simulink model "Main_bikesim_backup"  (R2025a)
settings: Solver=FixedStepAuto  StartTime=0.0  StopTime=inf  FixedStep=0.0005
values from neighbouring files (symbols this model uses):
  A_d = permute(A_d,[1,3,2])    [Main_sim.m]    (also in Startup_labview_v2.m; sensor_error_test_sequence.m = (eye(size(A))+Ts*A))
  Ad_t = eye(1)+Ts*A_t    [Main_sim.m]    (also in Startup_labview_v2.m = (eye(size(A_t))+Ts*A_t))
  B_d = zeros(V_n,7,1)    [Main_sim.m]    (also in Startup_labview_v2.m; sensor_error_test_sequence.m = Ts*B)
  badGPS = 0    [Main_sim.m]
  Bd_t = B_t*Ts    [Main_sim.m]    (also in Startup_labview_v2.m)
  bike_model = 1    [Main_sim.m]
  bike_params = LoadBikeParameters(bike)    [Compare_real_to_sim.m]    (also in MPC_Data_train.m = LoadBikeParameters("green"); Main_sim.m; Startup_labview_v2.m; sensor_error_test_sequence.m)
  C = mpc_outer_params.Cd    [MPC_Data_train.m]    (also in Main_sim.m = permute(C,[1,3,2]); Startup_labview_v2.m = permute(C,[1,3,2]); fromIMU2trajectory.m = (W_roll * W_roll.') / max(1, size(W_roll,2)); sensor_data_check.m = (W_roll * W_roll.') / max(1, size(W_roll,2)))
  C_t = zeros(V_n,1)    [Main_sim.m]    (also in Startup_labview_v2.m)
  counter = zeros(V_n,1)    [Main_sim.m]    (also in Startup_labview_v2.m; sensor_error_test_sequence.m = 9)
  D = mpc_outer_params.Dd    [MPC_Data_train.m]    (also in Main_sim.m = zeros(V_n,7,1); Startup_labview_v2.m = zeros(V_n,7,1))
  D_t = zeros(V_n,1)    [Main_sim.m]    (also in Startup_labview_v2.m)
  e1_max = abs(-k2*e2_max/k1)    [Startup_labview_v2.m]
  friction_coefficient = 0.004    [Main_sim.m]
  gg = 9.81    [Main_sim.m]    (also in Startup_labview_v2.m)
  hor_dis = 5    [Main_sim.m]
  I_balancing_outer = 0.0    (= 0)    [Main_sim.m]    (also in Startup_labview_v2.m; sensor_error_test_sequence.m)
  indoor = 0    [Main_sim.m]
  initial_state_estimate = initial_state    [Main_sim.m]    (also in sensor_error_test_sequence.m)
  interpolation = 0    [Main_sim.m]
  k1 = K(1)    [Startup_labview_v2.m]
  k2 = K(2)    [Startup_labview_v2.m]
  K_GPS = permute(K_GPS,[1,3,2])    [Main_sim.m]    (also in Startup_labview_v2.m)
  K_noGPS = permute(K_noGPS,[1,3,2])    [Main_sim.m]    (also in Startup_labview_v2.m)
  mpc_outer_params =     [MPC_params_train.mat]    (also in Main_sim.m = struct(); mpc_outer_params.mat)
  P_balancing_inner = 3.5    [Main_sim.m]    (also in Startup_labview_v2.m; sensor_error_test_sequence.m)
  P_balancing_outer = 3.75    [Main_sim.m]    (also in Startup_labview_v2.m; sensor_error_test_sequence.m)
  Psiref = [Psiref(1); Psiref]    [ReferenceGenerator.m]    (also in differenttest.m = [atan2(Yref(2)-Yref(1), Xref(2)-Xref(1)); differenttest_Simon.m = [psi(1); psi])
  ref_dis = 1    [Main_sim.m]    (also in differenttest.m = 0.1; differenttest_Simon.m = 0.1)
  T = [ 1,  sin(phi)*tan(th),  cos(phi)*tan(th) ... (first row only)    [Copy_of_fromIMU2trajectory.m]    (also in Main_sim.m = TransMatrix(bike_params); fromIMU2trajectory.m; sensor_error_test_sequence.m = Rz*Ry*Rx; shorttrajectory.m = table(Xref, Yref, Psiref, Vref, t, 'VariableNames', {'Xref',)
  t_ref = linspace(0, (lL-1)/Vref_test, lL)'    [differenttest.m]    (also in differenttest_Simon.m)
  Ts = 0.01    [Main_sim.m]    (also in Startup_labview_v2.m; sensor_error_test_sequence.m)
  V = round(V,1)    [Main_sim.m]    (also in Startup_labview_v2.m)
  v_init = Vref(1)    [Main_sim.m]    (also in Startup_labview_v2.m)
  Vref = zeros(length(Xref), 1)    [Refgeneration_test.m]    (also in differenttest_Simon.m = Vref_test * ones(N_line, 1))
  vv = 2    [Main_sim.m]    (also in Refgeneration.m = table_ref.v)
  Xref = [Xref;Xref2]    [ReferenceGenerator.m]    (also in concatenate.m; differenttest.m = interp1(cumulative_distance, x, equal_distances)'; differenttest_Simon.m = interp1(s, x_path, s_eq, 'linear')')
  Yref = [Yref;Yref2]    [ReferenceGenerator.m]    (also in concatenate.m; differenttest.m = interp1(cumulative_distance, y, equal_distances)'; differenttest_Simon.m = interp1(s, y_path, s_eq, 'linear')')
undefined symbols (not defined in the file or in its folder): initial_state, MPC_Ts, pert_deltadot_state, pert_deltadot_state_fun, pert_phidot_state, pert_phidot_state_fun
libraries: simulink x10, slpidlib x4, matrix_library x1, eeGeneralControl x1
(part 2 of 3)

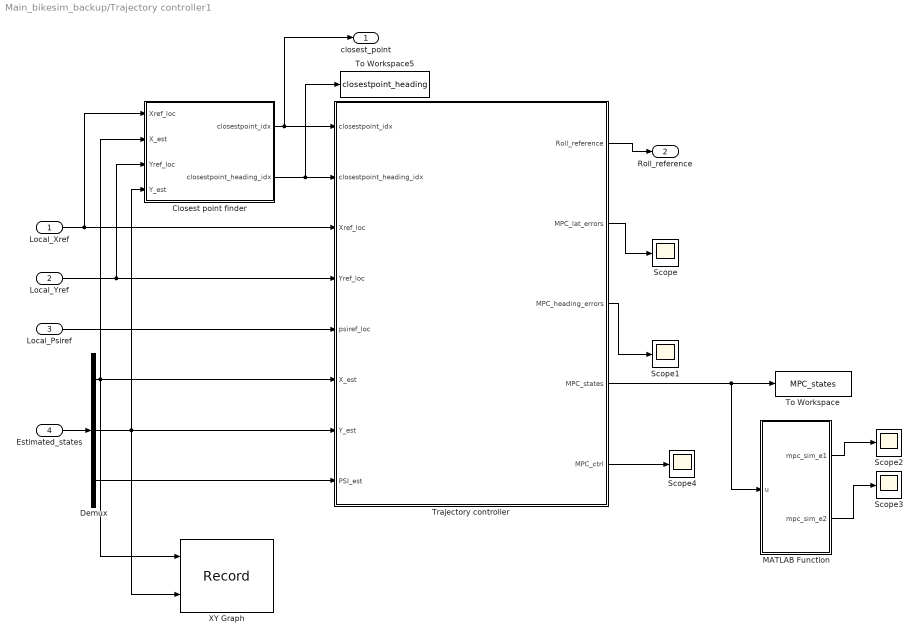
== system Main_bikesim_backup/Trajectory controller1 ==
  Local_Xref : Inport
  Local_Yref : Inport  Port=2
  Local_Psiref : Inport  Port=3
  Estimated_states : Inport  Port=4
  Closest point finder : MATLAB Function  TreatAsAtomicUnit=on
  Demux : Demux  Outputs=3
  MATLAB Function : MATLAB Function  TreatAsAtomicUnit=on
  Scope{,1..4} (5 alike) : Scope
      Scope settings: ActiveDisplayYMinimum=-10.323052116626126  ActiveDisplayYMaximum=2.50520359067044  DataLoggingVariableName=ScopeData21
      Scope1 settings: ActiveDisplayYMinimum=-2.3069490270114361  ActiveDisplayYMaximum=0.25967766677403764  DataLoggingVariableName=ScopeData22
      Scope2 settings: ActiveDisplayYMinimum=-0.54382498124419365  ActiveDisplayYMaximum=0.057362051727919812  DataLoggingVariableName=ScopeData28
      Scope3 settings: ActiveDisplayYMinimum=-0.21677334939399687  ActiveDisplayYMaximum=0.018061249921101648  DataLoggingVariableName=ScopeData29
      Scope4 settings: ActiveDisplayYMinimum=-0.43633231299858333  ActiveDisplayYMaximum=0.436332312998583  DataLoggingVariableName=ScopeData30
  To Workspace : ToWorkspace  VariableName=MPC_states  SaveFormat=Timeseries  SampleTime=-1
  To Workspace5 : ToWorkspace  VariableName=closestpoint_heading  SaveFormat=Timeseries  SampleTime=-1
  Trajectory controller : MATLAB Function  TreatAsAtomicUnit=on
  XY Graph : Record  NumPorts=2.0  FileSettingsInternal="{\"entries\":[{\"content\":{\"excelSettings\":{\"content\":{},\"type\":\"Streamout.ExcelSettings\"},\"parquetSettings\":{\"content\":{},\"type\":\"Streamout.ParquetSettings\"}},\"type\":\"Streamout.FileSettingStorage\",\"uuid\":\"\"}],\"packageUris\":[\"http:\\/\\/schema.mathworks.com\\/mf0\\/streamout_blocks\\/R2020a\"],\"version\":\"1.0\"}"  FrameSettings=[0, 0]  Layout=[1 1]  SignalsInternal="{\"entries\":[{\"content\":{\"signals\":[{\"content\":{\"blockPath\":[],\"dimensions\":[1],\"domain\":\"\",\"lineColor\":\"#edb120\",\"lineWidth\":2,\"port\":1,\"sid\":[\"\"],\"signalID\":1},\"type\":\"RecordBlkView.Signal\",\"uuid\":\"\"},{\"content\":{\"blockPath\":[],\"dimensions\":[1],\"domain\":\"\",\"lineColor\":\"#7e2f8e\",\"lineWidth\":2,\"port\":1,\"sid\":[\"\"],\"signalID\":2,\"signalName\":\"Add\"},\"type\":\"RecordBlkView.Signal\",\"uuid\":\"\"},{\"content\":{\"blockPath\":[],\"dimensions\":[7],\"domain\":\"\",\"hasChildren\":true,\"lineColor\":\"#7e2f8e\",\"lineWidth\":2,\"port\":1,\"sid\":[\"\"],\"signalID\":3},\"type\":\"RecordBlkView.Signal\",\"uuid\":\"\"},{\"content\":{\"blockPath\":[],\"channel\":[1],\"dimensions\":[7],\"domain\":\"\",\"lineColor\":\"#4dbeee\",\"lineWidth\":2,\"parentID\":3,\"port\":1,\"sid\":[\"\"],\"signalID\":4},\"type\":\"RecordBlkView.Signal\",\"uuid\":\"\"},{\"content\":{\"blockPath\":[],\"dimensions\":[1],\"domain\":\"\",\"lineColor\":\"#a2142f\",\"lineWidth\":2,\"port\":1,\"sid\":[\"\"],\"signalID\":5,\"signalName\":\"calculate pose_error based on projection point to reference point at time t\"},\"type\":\"RecordBlkView.Signal\",\"uuid\":\"\"},{\"content\":{\"blockPath\":[],\"dimensions\":[1],\"domain\":\"\",\"lineColor\":\"#139fff\",\"lineWidth\":2,\"port\":1,\"sid\":[\"\"],\"signalID\":6,\"signalName\":\"closest_point\"},\"type\":\"RecordBlkView.Signal\",\"uuid\":\"\"},{\"content\":{\"blockPath\":[],\"dimensions\":[7],\"domain\":\"\",\"hasChildren\":true,\"lineColor\":\"#139fff\",\"lineWidth\":2,\"port\":1,\"sid\":[\"\"],\"signalID\":7},\"type\":\"RecordBlkView.Signal\",\"uuid\":\"\"},{\"content\":{\"blockPath\":[],\"channel\":[1],\"dimensions\":[7],\"domain\":\"\",\"lineColor\":\"#b746ff\",\"lineWidth\":2,\"parentID\":7,\"port\":1,\"sid\":[\"\"],\"signalID\":8},\"type\":\"RecordBlkView.Signal\",\"uuid\":\"\"},{\"content\":{\"blockPath\":[],\"dimensions\":[7],\"domain\":\"\",\"hasChildren\":true,\"lineColor\":\"#b746ff\",\"lineWidth\":2,\"port\":1,\"sid\":[\"\"],\"signalID\":9},\"type\":\"RecordBlkView.Signal\",\"uuid\":\"\"},{\"content\":{\"blockPath\":[],\"channel\":[1],\"dimensions\":[7],\"domain\":\"\",\"lineColor\":\"#ff13a6\",\"lineWidth\":2,\"parentID\":9,\"port\":1,\"sid\":[\"\"],\"signalID\":10},\"type\":\"RecordBlkView.Signal\",\"uuid\":\"\"},{\"content\":{\"blockPath\":[],\"dimensions\":[1],\"domain\":\"\",\"lineColor\":\"#7e2f8e\",\"lineWidth\":2,\"port\":1,\"sid\":[\"\"],\"signalID\":11,\"signalName\":\"Trajectory controller:1\"},\"type\":\"RecordBlkView.Signal\",\"uuid\":\"\"},{\"content\":{\"blockPath\":[],\"dimensions\":[1],\"domain\":\"\",\"lineColor\":\"#77ac30\",\"lineWidth\":2,\"port\":1,\"sid\":[\"\"],\"signalID\":12,\"signalName\":\"Trajectory controller:2\"},\"type\":\"RecordBlkView.Signal\",\"uuid\":\"\"},{\"content\":{\"blockPath\":[],\"dimensions\":[1],\"domain\":\"\",\"lineColor\":\"#4dbeee\",\"lineWidth\":2,\"port\":1,\"sid\":[\"\"],\"signalID\":13,\"signalName\":\"Trajectory controller:6\"},\"type\":\"RecordBlkView.Signal\",\"uuid\":\"\"},{\"content\":{\"blockPath\":[],\"dimensions\":[1],\"domain\":\"\",\"lineColor\":\"#a2142f\",\"plots\":[ 1 ],\"port\":1,\"sid\":[\"\"],\"signalID\":14,\"signalName\":\"Demux:1\"},\"type\":\"RecordBlkView.Signal\",\"uuid\":\"\"},{\"content\":{\"blockPath\":[],\"dimensions\":[1],\"domain\":\"\",\"lineColor\":\"#139fff\",\"plots\":[ 1 ],\"port\":2,\"sid\":[\"\"],\"signalID\":15,\"signalName\":\"Demux:2\"},\"type\":\"RecordBlkView.Signal\",\"uuid\":\"\"},{\"content\":{\"blockPath\":[],\"dimensions\":[260],\"domain\":\"\",\"hasChildren\":true,\"lineColor\":\"#edb120\",\"lineWidth\":2,\"port\":1,\"sid\":[\"\"],\"signalID\":16,\"signalName\":\"Trajectory controller:4\"},\"type\":\"RecordBlkView.Signal\",\"uuid\":\"\"},{\"content\":{\"blockPath\":[],\"channel\":[1],\"dimensions\":[260],\"domain\":\"\",\"lineColor\":\"#d95319\",\"lineWidth\":2,\"parentID\":16,\"port\":1,\"sid\":[\"\"],\"signalID\":17,\"signalName\":\"Trajectory controller:4\"},\"type\":\"RecordBlkView.Signal\",\"uuid\":\"\"},{\"content\":{\"blockPath\":[],\"dimensions\":[1],\"domain\":\"\",\"lineColor\":\"#edb120\",\"lineWidth\":2,\"port\":1,\"sid\":[\"\"],\"signalID\":18,\"signalName\":\"Closest point finder:2\"},\"type\":\"RecordBlkView.Signal\",\"uuid\":\"\"},{\"content\":{\"blockPath\":[],\"dimensions\":[1],\"domain\":\"\",\"lineColor\":\"#7e2f8e\",\"lineWidth\":2,\"port\":1,\"sid\":[\"\"],\"signalID\":19},\"type\":\"RecordBlkView.Signal\",\"uuid\":\"\"},{\"content\":{\"blockPath\":[],\"dimensions\":[7],\"domain\":\"\",\"hasChildren\":true,\"lineColor\":\"#a2142f\",\"lineWidth\":2,\"port\":1,\"sid\":[\"\"],\"signalID\":20,\"signalName\":\"Mux\"},\"type\":\"RecordBlkView.Signal\",\"uuid\":\"\"},{\"content\":{\"blockPath\":[],\"channel\":[1],\"dimensions\":[7],\"domain\":\"\",\"lineColor\":\"#4dbeee\",\"lineWidth\":2,\"parentID\":20,\"port\":1,\"sid\":[\"\"],\"signalID\":21,\"signalName\":\"Mux\"},\"type\":\"RecordBlkView.Signal\",\"uuid\":\"\"},{\"content\":{\"blockPath\":[],\"dimensions\":[7],\"domain\":\"\",\"hasChildren\":true,\"lineColor\":\"#ff6929\",\"lineWidth\":2,\"port\":1,\"sid\":[\"\"],\"signalID\":22,\"signalName\":\"From10\"},\"type\":\"RecordBlkView.Signal\",\"uuid\":\"\"},{\"content\":{\"blockPath\":[],\"channel\":[1],\"dimensions\":[7],\"domain\":\"\",\"lineColor\":\"#139fff\",\"lineWidth\":2,\"parentID\":22,\"port\":1,\"sid\":[\"\"],\"signalID\":23,\"signalName\":\"From10\"},\"type\":\"RecordBlkView.Signal\",\"uuid\":\"\"},{\"content\":{\"blockPath\":[],\"dimensions\":[1],\"domain\":\"\",\"lineColor\":\"#a2142f\",\"lineWidth\":2,\"port\":1,\"sid\":[\"\"],\"signalID\":24,\"signalName\":\"From11\"},\"type\":\"RecordBlkView.Signal\",\"uuid\":\"\"},{\"content\":{\"blockPath\":[],\"dimensions\":[1],\"domain\":\"\",\"lineColor\":\"#139fff\",\"lineWidth\":2,\"port\":1,\"sid\":[\"\"],\"signalID\":25,\"signalName\":\"From12\"},\"type\":\"RecordBlkView.Signal\",\"uuid\":\"\"},{\"content\":{\"blockPath\":[],\"dimensions\":[1],\"domain\":\"\",\"lineColor\":\"#ff6929\",\"lineWidth\":2,\"port\":1,\"sid\":[\"\"],\"signalID\":26,\"signalName\":\"From13\"},\"type\":\"RecordBlkView.Signal\",\"uuid\":\"\"},{\"content\":{\"blockPath\":[],\"dimensions\":[1],\"domain\":\"\",\"lineColor\":\"#ff6929\",\"lineWidth\":2,\"port\":1,\"sid\":[\"\"],\"signalID\":27,\"signalName\":\"From17\"},\"type\":\"RecordBlkView.Signal\",\"uuid\":\"\"},{\"content\":{\"blockPath\":[],\"dimensions\":[1],\"domain\":\"\",\"lineColor\":\"#b746ff\",\"lineWidth\":2,\"port\":1,\"sid\":[\"\"],\"signalID\":28,\"signalName\":\"From18\"},\"type\":\"RecordBlkView.Signal\",\"uuid\":\"\"},{\"content\":{\"blockPath\":[],\"dimensions\":[1],\"domain\":\"\",\"lineColor\":\"#64d413\",\"lineWidth\":2,\"port\":1,\"sid\":[\"\"],\"signalID\":29,\"signalName\":\"From19\"},\"type\":\"RecordBlkView.Signal\",\"uuid\":\"\"},{\"content\":{\"blockPath\":[],\"dimensions\":[1],\"domain\":\"\",\"lineColor\":\"#ff13a6\",\"lineWidth\":2,\"port\":1,\"sid\":[\"\"],\"signalID\":30,\"signalName\":\"From20\"},\"type\":\"RecordBlkView.Signal\",\"uuid\":\"\"},{\"content\":{\"blockPath\":[],\"dimensions\":[20],\"domain\":\"\",\"lineColor\":\"#fe330a\",\"lineWidth\":2,\"port\":1,\"sid\":[\"\"],\"signalID\":31,\"signalName\":\"From21\"},\"type\":\"RecordBlkView.Signal\",\"uuid\":\"\"},{\"content\":{\"blockPath\":[],\"dimensions\":[20],\"domain\":\"\",\"lineColor\":\"#22b573\",\"lineWidth\":2,\"port\":1,\"sid\":[\"\"],\"signalID\":32,\"signalName\":\"From22\"},\"type\":\"RecordBlkView.Signal\",\"uuid\":\"\"},{\"content\":{\"blockPath\":[],\"dimensions\":[1],\"domain\":\"\",\"lineColor\":\"#0072bd\",\"lineWidth\":2,\"port\":1,\"sid\":[\"\"],\"signalID\":33,\"signalName\":\"From5\"},\"type\":\"RecordBlkView.Signal\",\"uuid\":\"\"},{\"content\":{\"blockPath\":[],\"dimensions\":[7],\"domain\":\"\",\"hasChildren\":true,\"lineColor\":\"#a2142f\",\"lineWidth\":2,\"port\":1,\"sid\":[\"\"],\"signalID\":34,\"signalName\":\"From7\"},\"type\":\"RecordBlkView.Signal\",\"uuid\":\"\"},{\"content\":{\"blockPath\":[],\"channel\":[1],\"dimensions\":[7],\"domain\":\"\",\"lineColor\":\"#edb120\",\"lineWidth\":2,\"parentID\":34,\"port\":1,\"sid\":[\"\"],\"signalID\":35,\"signalName\":\"From7\"},\"type\":\"RecordBlkView.Signal\",\"uuid\":\"\"},{\"content\":{\"blockPath\":[],\"dimensions\":[7],\"domain\":\"\",\"hasChildren\":true,\"lineColor\":\"#ff6929\",\"lineWidth\":2,\"port\":1,\"sid\":[\"\"],\"signalID\":36,\"signalName\":\"From8\"},\"type\":\"RecordBlkView.Signal\",\"uuid\":\"\"},{\"content\":{\"blockPath\":[],\"channel\":[1],\"dimensions\":[7],\"domain\":\"\",\"lineColor\":\"#77ac30\",\"lineWidth\":2,\"parentID\":36,\"port\":1,\"sid\":[\"\"],\"signalID\":37,\"signalName\":\"From8\"},\"type\":\"RecordBlkView.Signal\",\"uuid\":\"\"},{\"content\":{\"blockPath\":[],\"dimensions\":[1],\"domain\":\"\",\"lineColor\":\"#4dbeee\",\"lineWidth\":2,\"port\":1,\"sid\":[\"\"],\"signalID\":38,\"signalName\":\"From9\"},\"type\":\"RecordBlkView.Signal\",\"uuid\":\"\"}]},\"type\":\"RecordBlkView.InputSignals\",\"uuid\":\"\"}],\"packageUris\":[\"http:\\/\\/schema.mathworks.com\\/mf0\\/streamout_blocks\\/R2020a\"],\"version\":\"1.0\"}"  VisualizationBindings="{\"xyplotplugin\":{\"info\":[{\"series\":[{\"bindingParametersList\":[{\"parameter\":\"X-Axis\",\"signalID\":14,\"signalName\":\"Demux:1\"},{\"parameter\":\"Y-Axis\",\"signalID\":15,\"signalName\":\"Demux:2\"}],\"seriesID\":0}],\"subplotID\":1}]}}"  CompatibilityTag=XY
  closest_point : Outport
  Roll_reference : Outport  Port=2
  wires:
  Estimated_states/1 -> Demux/1
  Local_Xref/1 -> Closest point finder/1(Xref_loc), Trajectory controller/3(Xref_loc)
  Local_Psiref/1 -> Trajectory controller/5(psiref_loc)
  Demux/2 -> XY Graph/2, Closest point finder/4(Y_est), Trajectory controller/7(Y_est)
  Local_Yref/1 -> Closest point finder/3(Yref_loc), Trajectory controller/4(Yref_loc)
  Demux/1 -> XY Graph/1, Closest point finder/2(X_est), Trajectory controller/6(X_est)
  Closest point finder/1(closestpoint_idx) -> closest_point/1, Trajectory controller/1(closestpoint_idx)
  Closest point finder/2(closestpoint_heading_idx) -> To Workspace5/1, Trajectory controller/2(closestpoint_heading_idx)
  Demux/3 -> Trajectory controller/8(PSI_est)
  Trajectory controller/2(MPC_lat_errors) -> Scope/1
  Trajectory controller/3(MPC_heading_errors) -> Scope1/1
  Trajectory controller/1(Roll_reference) -> Roll_reference/1
  Trajectory controller/4(MPC_states) -> MATLAB Function/1(u), To Workspace/1
  MATLAB Function/1(mpc_sim_e1) -> Scope2/1
  MATLAB Function/2(mpc_sim_e2) -> Scope3/1
  Trajectory controller/5(MPC_ctrl) -> Scope4/1

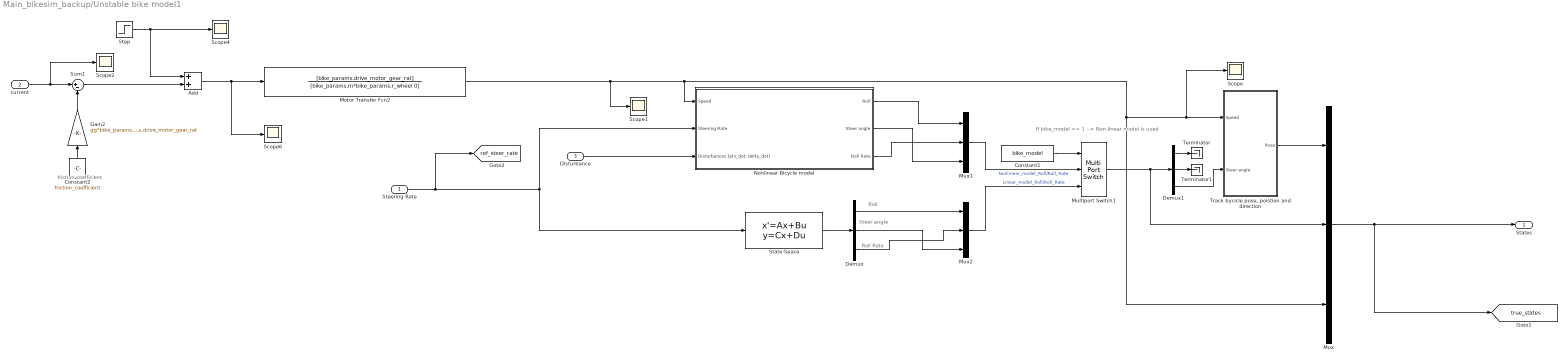
== system Main_bikesim_backup/Unstable bike model1 ==
  note: Steer angle
  note: Roll Rate
  note: Roll
  note: If bike_model == 1 --> Non-linear model is used
  note: friction coefficient
  Steering Rate : Inport
  current : Inport  Port=2
  Disturbance : Inport  Port=3
  Add : Sum
  Constant1 : Constant  Value=bike_model
  Constant2 : Constant  Value=friction_coefficient
  Demux : Demux  Outputs=3
  Demux1 : Demux  Outputs=3
  Gain2 : Gain  Gain=gg*bike_params.m*bike_params.r_wheel/bike_params.drive_motor_gear_rat
  Motor Transfer Fcn2 : TransferFcn  Numerator=[bike_params.drive_motor_gear_rat]  Denominator=[bike_params.m*bike_params.r_wheel 0]
  Multiport Switch1 : MultiPortSwitch  Inputs=2  SaturateOnIntegerOverflow=off  InputSameDT=off
  Mux : Mux  Inputs=3
  Mux1 : Mux  Inputs=3
  Mux2 : Mux  Inputs=3
  Nonlinear Bicycle model : Subsystem
  Scope{,1..2,4,6} (5 alike) : Scope
      Scope settings: ActiveDisplayYMinimum=-14.800391636195144  ActiveDisplayYMaximum=2.1206123892114217  DataLoggingVariableName=ScopeData4
      Scope1 settings: ActiveDisplayYMinimum=1  ActiveDisplayYMaximum=3  DataLoggingVariableName=ScopeData2
      Scope2 settings: ActiveDisplayYMinimum=-107.24515658734754  ActiveDisplayYMaximum=16.580853648483561  DataLoggingVariableName=ScopeData3
      Scope4 settings: ActiveDisplayYMinimum=-0.125  ActiveDisplayYMaximum=1.125  DataLoggingVariableName=ScopeData5
      Scope6 settings: ActiveDisplayYMinimum=-107.26411377256493  ActiveDisplayYMaximum=16.561896463266169
  State-Space : StateSpace  A=[0 0 1; 0 0 0 ; gg/bike_params.h (vv^2/bike_params.h-(gg*bike_params.lr*bike_params.c/(bike_params.h^2*(bike_params.lr+bike_params.lf))))*sin(bike_params.lambda) 0]  B=[0; 1 ; bike_params.lr*vv/((bike_params.lr+bike_params.lf)*bike_params.h)]  C=[1 0 0; 0 1 0 ; 0 0 1]  D=[0;0;0]  InitialCondition=[0; 0 ; 0]
  Step : Step  Time=10  After=0  SampleTime=5
  Sum1 : Sum  Inputs=|+-
  Terminator : Terminator
  Terminator1 : Terminator
  "Track bycicle pose, poistion and direction" : Subsystem
  States : Outport
  tag scope: ref_steer_rate=global, true_states=global
  wires:
  Steering Rate/1 -> State-Space/1, Nonlinear Bicycle model/2(Steering Rate), [ref_steer_rate]
  Nonlinear Bicycle model/3(Roll Rate) -> Mux1/2
  Nonlinear Bicycle model/2(Steer angle) -> Mux1/3
  Demux/1 -> Mux2/1
  Demux/3 -> Mux2/2
  Mux1/1 -> Multiport Switch1/2  "Nonlinear_model_Roll/Roll_Rate"
  Mux2/1 -> Multiport Switch1/3  "Linear_model_Roll/Roll_Rate"
  Constant1/1 -> Multiport Switch1/1
  Disturbance/1 -> Nonlinear Bicycle model/3(Disturbances (phi_dot; delta_dot))
  "Track bycicle pose, poistion and direction"/1(Pose) -> Mux/1
  Mux/1 -> States/1, [true_states]
  Nonlinear Bicycle model/1(Roll) -> Mux1/1
  State-Space/1 -> Demux/1
  Demux/2 -> Mux2/3
  Multiport Switch1/1 -> Mux/2, Demux1/1
  Demux1/3 -> "Track bycicle pose, poistion and direction"/2(Steer angle)
  Demux1/1 -> Terminator/1
  Demux1/2 -> Terminator1/1
  Constant2/1 -> Gain2/1
  Gain2/1 -> Sum1/2
  Sum1/1 -> Add/2
  Motor Transfer Fcn2/1 -> Scope1/1, Mux/3, Scope/1, "Track bycicle pose, poistion and direction"/1(Speed), Nonlinear Bicycle model/1(Speed)
  Step/1 -> Add/1, Scope4/1
  current/1 -> Scope2/1, Sum1/1
  Add/1 -> Motor Transfer Fcn2/1, Scope6/1

== system Main_bikesim_backup/Sensors1/Constant disturbances ==
  note: Apply the constant noise after 8sec
  Noise Channel : Inport
  Clock : Clock
  Constant4 : Constant  Value=[1 0.5 -0.2 0.2 0.1 0.02 0.3]'
  Constant7 : Constant  Value=[ 0 0 0 0 0 0 0]
  Create Diagonal Matrix : matrix_library/Create Diagonal Matrix
      settings: LibrarySourceBlock=|
      | simulink/Matrix
      | Operations/Create Diagonal
      | Matrix
  Matrix Multiply : Product  Multiplication=Matrix(*)
  Switch : Switch  Criteria=u2 > Threshold  Threshold=8  SaturateOnIntegerOverflow=off  InputSameDT=off
  Noise : Outport
  wires:
  Create Diagonal Matrix/1 -> Matrix Multiply/1
  Constant7/1 -> Switch/3
  Matrix Multiply/1 -> Switch/1
  Clock/1 -> Switch/2
  Constant4/1 -> Matrix Multiply/2
  Switch/1 -> Noise/1
  Noise Channel/1 -> Create Diagonal Matrix/1

== system Main_bikesim_backup/Sensors1/Subsystem ==
  X_coordinate : Inport
  Clock : Clock
  Gain1 : Gain  Gain=badGPS
  Memory : Memory
  Switch : Switch  Criteria=u2 > Threshold  SaturateOnIntegerOverflow=off  InputSameDT=off
  X_coordinate from GPS : Outport
  wires:
  Memory/1 -> Switch/1
  Clock/1 -> Gain1/1
  Switch/1 -> X_coordinate from GPS/1, Memory/1
  Gain1/1 -> Switch/2
  X_coordinate/1 -> Switch/3

== system Main_bikesim_backup/Sensors1/Subsystem1 ==
  Y_coordinate : Inport
  Clock : Clock
  Gain1 : Gain  Gain=badGPS
  Memory : Memory
  Switch : Switch  Criteria=u2 > Threshold  SaturateOnIntegerOverflow=off  InputSameDT=off
  Y_coordinate from GPS : Outport
  wires:
  Y_coordinate/1 -> Switch/3
  Gain1/1 -> Switch/2
  Switch/1 -> Memory/1, Y_coordinate from GPS/1
  Clock/1 -> Gain1/1
  Memory/1 -> Switch/1

== system Main_bikesim_backup/Unstable bike model1/Nonlinear Bicycle model ==
  Speed : Inport
  Steering Rate : Inport  Port=2
  Disturbances (phi_dot; delta_dot) : Inport  Port=3
  Demux : Demux  Outputs=3
  Integrator2 : Integrator  InitialCondition=[initial_state.roll ; initial_state.steering ; initial_state.roll_rate]
  MATLAB Function : MATLAB Function  TreatAsAtomicUnit=on
  Real Bike Parameters : Constant  Value=[gg bike_params.h bike_params.lr bike_params.lf bike_params.lambda bike_params.c bike_params.m bike_params.IMU_height bike_params.Xgps bike_params.Ygps bike_params.Hgps]  SampleTime=Ts
  Roll : Outport  VectorParamsAs1DForOutWhenUnconnected=off
  Steer angle : Outport  Port=2  VectorParamsAs1DForOutWhenUnconnected=off
  Roll Rate : Outport  Port=3  VectorParamsAs1DForOutWhenUnconnected=off
  wires:
  Steering Rate/1 -> MATLAB Function/2(Steering_rate)
  Disturbances (phi_dot; delta_dot)/1 -> MATLAB Function/4(disturbances)
  Real Bike Parameters/1 -> MATLAB Function/5(bike_params)
  Speed/1 -> MATLAB Function/3(Speed)
  Demux/1 -> Roll/1  "Roll Angle"
  Demux/3 -> Roll Rate/1  "Roll Rate"
  Demux/2 -> Steer angle/1  "Steering Angle"
  Integrator2/1 -> MATLAB Function/1(States), Demux/1
  MATLAB Function/1(xdot) -> Integrator2/1

== system Main_bikesim_backup/Unstable bike model1/Track bycicle pose, poistion and direction ==
  Speed : Inport
  Steer angle : Inport  Port=2
  Constant : Constant  Value=[bike_params.lr bike_params.lf bike_params.lambda]
  Derivative of positions : MATLAB Function  TreatAsAtomicUnit=on
  Integrator with Wrapped State (between -pi & pi) : eeGeneralControl/Integrator with Wrapped State (Discrete or Continuous)  LabelModeActiveChoice=Discrete  WrappedStateUpperValue=pi  WrappedStateLowerValue=-pi  x0=initial_state_estimate.heading  Ts=Ts
  Integrator1 : Integrator  InitialCondition=initial_state_estimate.x
  Integrator2 : Integrator  InitialCondition=initial_state_estimate.y
  MATLAB Function : MATLAB Function  TreatAsAtomicUnit=on
  Mux : Mux  Inputs=3
  Pose : Outport
  tag scope: Xposition4debug=global
  wires:
  Derivative of positions/2(Ydot) -> Integrator2/1  "Ydot"
  Steer angle/1 -> MATLAB Function/2(steer_angle)
  Integrator2/1 -> Mux/2
  Mux/1 -> Pose/1
  Derivative of positions/1(Xdot) -> Integrator1/1  "Xdot"
  Speed/1 -> MATLAB Function/1(Speed), Derivative of positions/1(Speed)
  Integrator1/1 -> [Xposition4debug], Mux/1
  MATLAB Function/1(beta) -> Derivative of positions/2(beta)
  Constant/1 -> MATLAB Function/3(bike_params)
  MATLAB Function/2(psi_dot) -> Integrator with Wrapped State (between -pi & pi)/1
  Integrator with Wrapped State (between -pi & pi)/1 -> Derivative of positions/3(psi), Mux/3

== matlab function Main_bikesim_backup/current position on the trajectory, projection from estimated position ==
  settings: updateMethod=DISCRETE  sampleTime=Ts
  data: Xest input; Yest input; Xref_loc input; Yref_loc input; closest_point input; X_projection output; Y_projection output; closest2closestplus1 output
function [X_projection, Y_projection,closest2closestplus1] = Closest2estOntoClosest2interp(Xest, Yest, Xref_loc, Yref_loc, closest_point)
    
    % Construct vector closest2est
    closest2est = [Xest - Xref_loc(closest_point), Yest - Yref_loc(closest_point)];

    % Construct vector closest2closestplus1
    closest2closestplus1 = [Xref_loc(closest_point+1) - Xref_loc(closest_point), Yref_loc(closest_point+1) - Yref_loc(closest_point)];

    % Calculate the dot product of closest2est and closest2closestplus1
    dot_product = dot(closest2est, closest2closestplus1);

    % Calculate the magnitude squared of closest2closestplus1
    closest2closestplus1_magnitude_squared = dot(closest2closestplus1, closest2closestplus1);

    % Calculate the projection_ratio
    projection_ratio = dot_product/closest2closestplus1_magnitude_squared;

    % Calculate the X coordinate of the projection point
    X_projection = Xref_loc(closest_point) +  projection_ratio*(Xref_loc(closest_point+1) - Xref_loc(closest_point));

    % Calculate the Y coordinate of the projection point
    Y_projection = Yref_loc(closest_point) +  projection_ratio*(Yref_loc(closest_point+1) - Yref_loc(closest_point));
end

== matlab function Main_bikesim_backup/Sensors1/MATLAB Function ==
  data: V parameter; C3 output; C parameter; Estimated_Velocity input; interpolation parameter
function C3=fcn(V, C, Estimated_Velocity, interpolation)
% Finding the index of closest and second closest velocities in the calculated velocity vector(in main.m) that corresponds to the
% gains and matrices based on our estimated velocity (i.e the estimated
% velocity is between these two closest V's)
    differences = abs(V - Estimated_Velocity);
    [~, index1] = min(differences);
    differences(index1)=inf;
    [~, index2] = min(differences);

% Implementing linear interpolation when estimated velocity is inside the
% range of minimum and maximum calculated velocity vector
if Estimated_Velocity<=max(V) & Estimated_Velocity>=min(V) & interpolation
    C1=C(index1,:,:);
    C2=C(index2,:,:);
    C1=squeeze(C1);
    C2=squeeze(C2);
    C3=C2*abs((Estimated_Velocity-V(index1))/(V(index1)-V(index2)))+C1*abs((Estimated_Velocity-V(index2))/(V(index1)-V(index2)));
    C3=C3';
    
% If no interpolation or the estimated velocity outside the velocity vector range, then take the closest velocity's gains and matrices
else


    C=C(index1,:,:);
    C3=squeeze(C);
    C3=C3';
end

== matlab function Main_bikesim_backup/Trajectory controller + closest_point selection1/Trajectory controller ==
  settings: updateMethod=DISCRETE  sampleTime=Ts
  data: closestpoint_idx_in input; closestpoint_idx_in output; e1 output; e2 output; Xref_loc input; Yref_loc input; psiref_loc input; X_est input; Y_est input; psi_est input; traj_control_params input; v input; Vest input; delta_ref output; delta_ref_psi output; D_psiref output; x input; x_dot output; Ad_t parameter; Bd_t parameter; C_t parameter; D_t parameter; V parameter; interpolation parameter
function [closestpoint_idx_in,e1,e2,delta_ref,delta_ref_psi,D_psiref,x_dot]= ...
    fcn(closestpoint_idx_in,Xref_loc,Yref_loc,psiref_loc,X_est,Y_est,psi_est,traj_control_params, ...
                                                                              v, Vest, x, Ad_t, Bd_t, C_t, D_t, V, interpolation)
%% calculations on a local part of the trajectory

% Unpack parameters, TODO use unpack...
%% qianlei 1023
% gg  = bike_params(1);
% lr = bike_params(2);
% lf = bike_params(3);
% lambda = bike_params(4);

k1 = traj_control_params(1);
k2 = traj_control_params(2);
e1_max = traj_control_params(3);

% Search for closest point --> Finding the closest point going forward. Stop searching once next distance increases
while (Xref_loc(closestpoint_idx_in,1)-X_est)^2 + (Yref_loc(closestpoint_idx_in,1)-Y_est)^2 >= (Xref_loc(closestpoint_idx_in+1,1)-X_est)^2+(Yref_loc(closestpoint_idx_in+1,1)-Y_est)^2  && closestpoint_idx_in <= length(Xref_loc)-2
    closestpoint_idx_in = closestpoint_idx_in+1;
end

% Select same closest point (for heading error and position error)
closestpoint_heading_idx = closestpoint_idx_in;

% Calculate X and Y distance from current location to selected closest
% point
dx = X_est - Xref_loc(closestpoint_idx_in,1);
dy = Y_est - Yref_loc(closestpoint_idx_in,1);

% Calculate difference in current heading and heading in reference point 
% And limit D_psiref  between pi and -pi
D_psiref = psiref_loc(closestpoint_idx_in+1,1)-psiref_loc(closestpoint_idx_in,1);
D_psiref = wrapToPi(D_psiref);
% if D_psiref>=pi
%     D_psiref=mod(D_psiref,-2*pi);
% end
% if D_psiref<=-pi
%     D_psiref=mod(D_psiref,2*pi);
% end

%IMPROVEMENT: implement an interpolation algoritm
% Calculate distence between point before closest point and current location
dist_true_previous = sqrt((Xref_loc(closestpoint_idx_in-1,1)-X_est)^2+(Yref_loc(closestpoint_idx_in-1,1)-Y_est)^2);
% Angle of line between previous closest point and current location
alpha_star = atan((Yref_loc(closestpoint_idx_in-1,1)-Y_est)/(Xref_loc(closestpoint_idx_in-1,1)-X_est));
% heading previous closest point - alpha star
alpha_projected_dist = alpha_star-psiref_loc(closestpoint_idx_in,1);
% the distance from the previous closest point to the projection of the bike on the trajectory
Projected_dist = abs(dist_true_previous*cos(alpha_projected_dist));

compared_dist = sqrt((Xref_loc(closestpoint_idx_in,1)-Xref_loc(closestpoint_idx_in-1,1))^2+(Yref_loc(closestpoint_idx_in,1)-Yref_loc(closestpoint_idx_in-1,1))^2);

% If bike passes closest point, the heading of the next point will be taken
if Projected_dist >= compared_dist
closestpoint_heading_idx = closestpoint_idx_in+1;
end

%calculate e1 and e2        
e1= dy*cos(psiref_loc(closestpoint_heading_idx,1)) - dx*sin(psiref_loc(closestpoint_heading_idx,1)); % this make e1 include "direction" automatically
e2= psi_est-psiref_loc(closestpoint_heading_idx,1); %calculate e2

% closest point on the local trajectory
ref_X=Xref_loc(closestpoint_idx_in,1);
ref_Y=Yref_loc(closestpoint_idx_in,1);
ref_psi=psiref_loc(closestpoint_heading_idx,1);

 % keep heading error should be between -pi 2 pi
e2 = wrapToPi(e2);
%e2=mod(e2+pi,2*pi)-pi;     

% Steering contribution from trajectory error
% delta_ref_error=-k1*sign(e1)*min(abs(e1),e1_max)-k2*e2;
delta_e1 = -k1*sign(e1)*min(abs(e1),e1_max);
delta_e2 =-k2*e2;
% delta_e1 = -2;
% delta_e2 = 0;
%delta_ref_error = delta_e1 + delta_e2;

% Steering contribution from trajectory error, ie feedback of trajectory
% error
delta_ref_error = -k1*sign(e1)*min(abs(e1),e1_max)-k2*e2;

% the following lines is a filtering of the reference direction, it is
% a speed dependent linear filter

% TODO is similar interpolations done on other places, for example in the
% Kalman filter_ If yes, check if a common function can be used and avoid
% doubling code

%calculate the time between psiref(idx,1) and psiref(idx+1,1)
dX=Xref_loc(closestpoint_idx_in+1,1)-ref_X;
dY=Yref_loc(closestpoint_idx_in+1,1)-ref_Y;
dis=sqrt(dX^2+dY^2);
Ts_psi=dis/v;

% Sample dpsiref
dpsiref=(D_psiref)/Ts_psi;


% Finding the index of closest and second closest velocities in the calculated velocity vector(in main.m) that corresponds to the
% gains and matrices based on our estimated velocity (i.e the estimated
% velocity is between these two closest V's)
differences = abs(V - Vest);
[~, index1] = min(differences);
differences(index1)=inf;
[~, index2] = min(differences);

% Implementing linear interpolation when estimated velocity is inside the
% range of minimum and maximum calculated velocity vector
if Vest<=max(V) & Vest>=min(V) & interpolation

    Ad_t1=Ad_t(index1,:);
    Ad_t2=Ad_t(index2,:);
    Ad_t=Ad_t2*abs((Vest-V(index1))/(V(index1)-V(index2)))+Ad_t1*abs((Vest-V(index2))/(V(index1)-V(index2)));
    Bd_t1=Bd_t(index1,:);
    Bd_t2=Bd_t(index2,:);
    Bd_t=Bd_t2*abs((Vest-V(index1))/(V(index1)-V(index2)))+Bd_t1*abs((Vest-V(index2))/(V(index1)-V(index2)));
    C_t1=C_t(index1,:);
    C_t2=C_t(index2,:);
    C_t=C_t2*abs((Vest-V(index1))/(V(index1)-V(index2)))+C_t1*abs((Vest-V(index2))/(V(index1)-V(index2)));
    D_t1=D_t(index1,:);
    D_t2=D_t(index2,:);
    D_t=D_t2*abs((Vest-V(index1))/(V(index1)-V(index2)))+D_t1*abs((Vest-V(index2))/(V(index1)-V(index2)));
    
% If no interpolation or the estimated velocity outside the velocity vector range, then take the closest velocity's gains and matrices
else
    Ad_t=Ad_t(index1,:);
    Bd_t=Bd_t(index1,:);
    C_t=C_t(index1,:);
    D_t=D_t(index1,:);
end


% Steering contribution from heading change
x_dot = Ad_t*x + Bd_t*dpsiref;
delta_ref_psi = (C_t*x + D_t*dpsiref); 
% delta_ref_psi = 0; 

% Total steering reference 
delta_ref = delta_ref_psi + delta_ref_error;

% limit steer angle between -pi/4 and pi/4
if delta_ref>=pi/4
    delta_ref=pi/4;
end

if delta_ref<=-pi/4
    delta_ref=-pi/4;
end

% % Transform steering reference into roll reference for balancing controller
% eff_delta_ref = delta_ref*sin(lambda);
% roll_ref = -1*atan(tan(eff_delta_ref)*(Vest^2/(lr+lf))/gg);

end

== matlab function Main_bikesim_backup/Trajectory controller/Closest point finder ==
  settings: updateMethod=DISCRETE  sampleTime=Ts
  data: Xref_loc input; closestpoint_idx output; X_est input; Yref_loc input; Y_est input; closestpoint_heading_idx output
function [closestpoint_idx, closestpoint_heading_idx] = fcn(Xref_loc, X_est, Yref_loc, Y_est)
% Each referencepoint has a location (X,Y) and a heading
% The heading is defined in the startup.m file as 'the heading where its coming from' 
% Second point in local reference is current selected closest point
closestpoint_idx=2;

% Search for closest point
% Finding the closest point going forward. Stop searching once next
% distance increases

while (Xref_loc(closestpoint_idx,1)-X_est)^2 + (Yref_loc(closestpoint_idx,1)-Y_est)^2 >= (Xref_loc(closestpoint_idx+1,1)-X_est)^2+(Yref_loc(closestpoint_idx+1,1)-Y_est)^2  && closestpoint_idx <= length(Xref_loc)-2
closestpoint_idx = closestpoint_idx+1;
end

% Select same closest point (for heading error and position error)
closestpoint_heading_idx = closestpoint_idx;

== matlab function Main_bikesim_backup/Sensors1/Define true sensor positions on the bike ==
  data: bike_params input; pose input; pose_corrected output
function pose_corrected  = fcn(bike_params, pose)
pose_corrected = pose;

gpsX = bike_params(1); % measured offset of GPS parallel to bike
gpsY = bike_params(2); % measured offset of GPS perpendicular to bike
gpsH = bike_params(3); % measured offset of GPS from ground to GPS

% define pose_l
pose_l = pose;

% Transform to local frame
    pose_l(1) =  pose(1) * cos(pose(3)) + pose(2) * sin(pose(3));
    pose_l(2) = -pose(1) * sin(pose(3)) + pose(2) * cos(pose(3)); 

% define actual positions of GPS 
% pose1 = difference in x in local frame
% pose2 = difference in y in local frame
    pose_l(1) = pose_l(1) + gpsX;
    pose_l(2) = pose_l(2) + gpsY + gpsH*sin(pose(4));

% define actual positions of IMU 


% Transform back to global frame
    pose(1) = pose_l(1) * cos(pose(3)) - pose_l(2) * sin(pose(3));
    pose(2) = pose_l(1) * sin(pose(3)) + pose_l(2) * cos(pose(3));

pose_corrected(1) = pose(1);
pose_corrected(2) = pose(2);

== matlab function Main_bikesim_backup/reference position at time t, interpolation of reference points  ==
  settings: updateMethod=DISCRETE  sampleTime=Ts
  data: vref_t output; Xref_t output; Yref_t output; Xref_loc input; Yref_loc input; t_ref_loc input; vref_loc input; t_now input
function [vref_t, Xref_t,Yref_t]= fcn(Xref_loc,Yref_loc,t_ref_loc,vref_loc,t_now) 
    
%disp(t_now)
%disp([Xref_loc Yref_loc t_ref_loc])
    % Find index point before the bike
    n = 1; 
    
    if t_now < t_ref_loc(1)
        disp('this should not happen, check reference point in position controller');
    end

    %% 
    while t_now >= t_ref_loc(n+1), n = n+1;end  
    
    % Calculate normalized time ratio between two reference points
    t_int=(t_now-t_ref_loc(n))/(t_ref_loc(n+1)-t_ref_loc(n)); 
       
    % X_ref position at t_now using linear interpolation between n and n+1
    Xref_t = Xref_loc(n)+t_int*(Xref_loc(n+1)-Xref_loc(n));   

    % Y_ref position at t_now using linear interpolation between n and n+1
    Yref_t = Yref_loc(n)+t_int*(Yref_loc(n+1)-Yref_loc(n));    

    % v_ref position at t_now using linear interpolation between n and n+1
    vref_t = vref_loc(n)+t_int*(vref_loc(n+1)-vref_loc(n));

end

== matlab function Main_bikesim_backup/State estimator1/Linearized Bicycle Model on Constant Velocity ==
  data: Est_States input; dot_delta input; y input; bike_params input; Est_states output; flag input; T parameter; indoor parameter; K_GPS parameter; K_noGPS parameter; V parameter; A_d parameter; B_d parameter; C parameter; D parameter; interpolation parameter
function Est_states  = fcn(Est_States, dot_delta, y, bike_params, flag, T, indoor, K_GPS, K_noGPS, V, A_d, B_d, C, D, interpolation)
% description 
% Inputs
%   Est_States := [X Y psi phi phi_dot delta v] are global at time t 
%   dot_delta_e := effective steering rate
%   y := measurement vector
%   bike_params := vector of bike parameters + gravity
%   flag := [0-1] increasing counter reseted at 1. When flag == 0 means
%           that GPS measurement is available
%   indoor := it's 1 when you want to run the bike indoor
%   K_GPS := Computed state_feedback gain including GPS meas
%   K_noGPS := Computed state_feedback gain excluding GPS meas
%
% Outputs
%   Est_states : = [X Y psi phi phi_dot delta v] global at time t+1

% PROBABLY IS BETTER IF WE CHANGE THE NAME OF Est_states AND Est_States

% Transform the states to local frame 
    Est_States_l = zeros(7,1);
    
    Est_States_l(1) = Est_States(1) * cos(Est_States(3)) + Est_States(2) * sin(Est_States(3));
    Est_States_l(2) = -Est_States(1) * sin(Est_States(3)) + Est_States(2) * cos(Est_States(3));
    Est_States_l(3) = 0;        % direction of bike is aligned with X local frame
    Est_States_l(4) = Est_States(4);
    Est_States_l(5) = Est_States(5);
    Est_States_l(6) = Est_States(6);
    Est_States_l(7) = Est_States(7);

% Transform measurements to local frame
    y_l = zeros(size(y));

    y_l(1) = y(1) * cos(Est_States(3)) + y(2) * sin(Est_States(3));
    y_l(2) = -y(1) * sin(Est_States(3)) + y(2) * cos(Est_States(3)); 
    % y_l(3) = y(3);
    % y_l(4) = y(4);
    % y_l(5) = y(5);
    % y_l(6) = y(6);
    % y_l(7) = y(7);
    y_l(3:7) = y(3:7);

% Correct for parameter values/sensor positions
% The parameters/positions are measures by us (can differ from true values)
    X_gps_mod = bike_params(1);
    Y_gps_mod = bike_params(2);
    H_gps_mod = bike_params(3);
    
    y_l(1) = y_l(1) - X_gps_mod;
    y_l(2) = y_l(2) - Y_gps_mod - H_gps_mod*sin(Est_States(4));
    
% IMU correction
    raw_acc  = [0 y_l(3) 0];
    raw_gyro = [y_l(4) 0 y_l(5)];
    
% Apply the correction to the accelerometer measurement
    acc_corr = T*raw_acc';
    
% Apply the correction to the gyro measurement
    gyro_corr = T*raw_gyro';
% Results
    y_l(3) =acc_corr(2) ;
    y_l(4) =gyro_corr(1) ;
    y_l(5) =gyro_corr(3) ;
    % 
% % Continuous Time update in local frame TODO: x(t+1) = (I+A delta_T)h_hat(t)
    %     states_dot = zeros(7,1);
    %     
    %     states_dot(1) = Est_States(7);
    %     states_dot(2) = v * (Est_States_l(3) + (lr/(lr+lf))*Est_States(6) );
    %     states_dot(3) = (v/(lr+lf)) * Est_States(6);
    %     states_dot(4) = Est_States(5);
    %     states_dot(5) =(g/h)*Est_States(4) + ((lr*v)/((lr+lf)*h))*sin(lambda)*dot_delta + ((h*v^2-g*lr*c)/((lr+lf)*h^2))*sin(lambda)*Est_States(6);
    %     states_dot(6) = dot_delta;
    %     states_dot(7) = 0;
    % 
% % Discrete time update in local 
    %     Est_States_l = Est_States_l + states_dot * Ts; 
    
% % C identity is used to see if the code runs
    %     sen = zeros(6,1);
    %     sen(1)      = States_l(1);  
    %     sen(2)      = States_l(2);
    %     %sen(3)      = States_l(3);
    %     sen(3)      = States_l(4);
    %     sen(4)      = States_l(5);
    %     sen(5)      = States_l(6);
    %     sen(6)      = States_l(7);
    
% % Transform measurements into local frame to see if code runs
    %     meas_l = zeros(6,1);
    %     meas_l(1) = meas(1) * cos(States(3)) + meas(2) * sin(States(3));
    %     meas_l(2) = -meas(1) * sin(States(3)) + meas(2) * cos(States(3));
    %     meas_l(3) = 0;
    %     meas_l(3) = meas(3)-States(3);  
    %     meas_l(3) = meas(4);
    %     meas_l(4) = meas(5);
    %     meas_l(5) = meas(6);
    %     meas_l(6) = meas(7);
    %     meas_l(7) = meas(7);
%b3rbrgb

% Finding the index of closest and second closest velocities in the calculated velocity vector(in main.m) that corresponds to the
% gains and matrices based on our estimated velocity (i.e the estimated
% velocity is between these two closest V's)
    differences = abs(V - Est_States(7));
    [~, index1] = min(differences);
    differences(index1)=inf;
    [~, index2] = min(differences);

% Implementing linear interpolation when estimated velocity is inside the
% range of minimum and maximum calculated velocity vector
if Est_States(7)<=max(V) & Est_States(7)>=min(V) & interpolation

    K_GPS1=K_GPS(index1,:,:);
    K_GPS2=K_GPS(index2,:,:);
    K_GPS1=squeeze(K_GPS1);
    K_GPS2=squeeze(K_GPS2);
    K_GPS=K_GPS2*abs((Est_States(7)-V(index1))/(V(index1)-V(index2)))+K_GPS1*abs((Est_States(7)-V(index2))/(V(index1)-V(index2)));

    K_noGPS1=K_noGPS(index1,:,:);
    K_noGPS2=K_noGPS(index2,:,:);
    K_noGPS1=squeeze(K_noGPS1);
    K_noGPS2=squeeze(K_noGPS2);
    K_noGPS=K_noGPS2*abs((Est_States(7)-V(index1))/(V(index1)-V(index2)))+K_noGPS1*abs((Est_States(7)-V(index2))/(V(index1)-V(index2)));
   
    Ad1=A_d(index1,:,:);
    Ad2=A_d(index2,:,:);
    Ad1=squeeze(Ad1);
    Ad2=squeeze(Ad2);
    A_d=Ad2.*abs((Est_States(7)-V(index1))/(V(index1)-V(index2)))+Ad1*abs((Est_States(7)-V(index2))/(V(index1)-V(index2)));

    Bd1=B_d(index1,:,:);
    Bd2=B_d(index2,:,:);
    Bd1=squeeze(Bd1);
    Bd2=squeeze(Bd2);
    B_d=Bd2*abs((Est_States(7)-V(index1))/(V(index1)-V(index2)))+Bd1*abs((Est_States(7)-V(index2))/(V(index1)-V(index2)));

    C1=C(index1,:,:);
    C2=C(index2,:,:);
    C1=squeeze(C1);
    C2=squeeze(C2);
    C=C2*abs((Est_States(7)-V(index1))/(V(index1)-V(index2)))+C1*abs((Est_States(7)-V(index2))/(V(index1)-V(index2)));

    D1=D(index1,:,:);
    D2=D(index2,:,:);
    D1=squeeze(D1);
    D2=squeeze(D2);
    D=D2*abs((Est_States(7)-V(index1))/(V(index1)-V(index2)))+D1*abs((Est_States(7)-V(index2))/(V(index1)-V(index2)));

% If no interpolation or the estimated velocity outside the velocity vector range, then take the closest velocity's gains and matrices
else 
    K_GPS=K_GPS(index1,:,:);
    K_GPS=squeeze(K_GPS);

    K_noGPS=K_noGPS(index1,:,:);
    K_noGPS=squeeze(K_noGPS);

    A_d=A_d(index1,:,:);
    A_d=squeeze(A_d);
    B_d=B_d(index1,:,:);
    B_d=squeeze(B_d);
    C=C(index1,:,:);
    C=squeeze(C);
    D=D(index1,:,:);
    D=squeeze(D);
end
% Time update in local frame (from t to t+1)

    % Time update
     Est_States_l = A_d'*Est_States_l + B_d'*dot_delta;

    % Measurement update in local frame
     Est_states_l = zeros(7,1);

    % Sampling differentiation (Sensors rate 100Hz but GPS 10Hz)

    if flag == 0 && indoor == 0 % new GPS measurement and outdoor    
        K = K_GPS';

    else % no new GPS measurement or indoor    
        K = K_noGPS';
    end

% Measurement prediction
    y_pred = C'*Est_States_l + D'*dot_delta;

% Measurement update
    Est_states_l = Est_States_l + K * (y_l - y_pred);
    
    %Useless?
    % states_l = Kalman_gain * (meas_l - sen);
    % states_l(1) = States_l(1) + Kalman_gain(1,1) * (meas_l(1) - x_m) + Kalman_gain(1,2) * (meas_l(2) - y_m) + Kalman_gain(1,3) * (meas_l(3) - psi_m) + Kalman_gain(1,4) * (meas_l(4) - phi_m) + Kalman_gain(1,5) * (meas_l(5) - dot_phi_m) + Kalman_gain(1,6) * (meas_l(6) - delta_m) + Kalman_gain(1,7) * (meas_l(7) - v_m);
    % states_l(2) = States_l(2) + Kalman_gain(2,1) * (meas_l(1) - x_m) + Kalman_gain(2,2) * (meas_l(2) - y_m) + Kalman_gain(2,3) * (meas_l(3) - psi_m) + Kalman_gain(2,4) * (meas_l(4) - phi_m) + Kalman_gain(2,5) * (meas_l(5) - dot_phi_m) + Kalman_gain(2,6) * (meas_l(6) - delta_m) + Kalman_gain(2,7) * (meas_l(7) - v_m);
    % states_l(3) = States_l(3) + Kalman_gain(3,1) * (meas_l(1) - x_m) + Kalman_gain(3,2) * (meas_l(2) - y_m) + Kalman_gain(3,3) * (meas_l(3) - psi_m) + Kalman_gain(3,4) * (meas_l(4) - phi_m) + Kalman_gain(3,5) * (meas_l(5) - dot_phi_m) + Kalman_gain(3,6) * (meas_l(6) - delta_m) + Kalman_gain(3,7) * (meas_l(7) - v_m);
    % states_l(4) = States_l(4) + Kalman_gain(4,1) * (meas_l(1) - x_m) + Kalman_gain(4,2) * (meas_l(2) - y_m) + Kalman_gain(4,3) * (meas_l(3) - psi_m) + Kalman_gain(4,4) * (meas_l(4) - phi_m) + Kalman_gain(4,5) * (meas_l(5) - dot_phi_m) + Kalman_gain(4,6) * (meas_l(6) - delta_m) + Kalman_gain(4,7) * (meas_l(7) - v_m);
    % states_l(5) = States_l(5) + Kalman_gain(5,1) * (meas_l(1) - x_m) + Kalman_gain(5,2) * (meas_l(2) - y_m) + Kalman_gain(5,3) * (meas_l(3) - psi_m) + Kalman_gain(5,4) * (meas_l(4) - phi_m) + Kalman_gain(5,5) * (meas_l(5) - dot_phi_m) + Kalman_gain(5,6) * (meas_l(6) - delta_m) + Kalman_gain(5,7) * (meas_l(7) - v_m);
    % states_l(6) = States_l(6) + Kalman_gain(6,1) * (meas_l(1) - x_m) + Kalman_gain(6,2) * (meas_l(2) - y_m) + Kalman_gain(6,3) * (meas_l(3) - psi_m) + Kalman_gain(6,4) * (meas_l(4) - phi_m) + Kalman_gain(6,5) * (meas_l(5) - dot_phi_m) + Kalman_gain(6,6) * (meas_l(6) - delta_m) + Kalman_gain(6,7) * (meas_l(7) - v_m);
    % states_l(7) = States_l(7) + Kalman_gain(7,1) * (meas_l(1) - x_m) + Kalman_gain(7,2) * (meas_l(2) - y_m) + Kalman_gain(7,3) * (meas_l(3) - psi_m) + Kalman_gain(7,4) * (meas_l(4) - phi_m) + Kalman_gain(7,5) * (meas_l(5) - dot_phi_m) + Kalman_gain(7,6) * (meas_l(6) - delta_m) + Kalman_gain(7,7) * (meas_l(7) - v_m);

% Transform to global the local states at time t+1 after measurement update
    Est_states = zeros(7,1);
    Est_states(3) = Est_States(3) + Est_states_l(3);    % direction update global
    
% Change of Coordinates from local to global frame for  states 
    Est_states(1) = Est_states_l(1) * cos(Est_States(3)) - Est_states_l(2) * sin(Est_States(3));
    Est_states(2) = Est_states_l(1) * sin(Est_States(3)) + Est_states_l(2) * cos(Est_States(3));
    Est_states(4) = Est_states_l(4);
    Est_states(5) = Est_states_l(5);
    Est_states(6) = Est_states_l(6);
    Est_states(7) = Est_states_l(7);


    
% Heading angle between pi and -pi
    Est_states(3) = wrapToPi(Est_states(3));

end

== matlab function Main_bikesim_backup/calculate pose_error based on projection point to reference point at time t ==
  settings: updateMethod=DISCRETE  sampleTime=Ts
  data: pose_error output; Xref_t input; Yref_t input; X_projection input; Y_projection input; closest2closestplus1 input
function pose_error  = calculatePoseError(Xref_t, Yref_t, X_projection, Y_projection, closest2closestplus1)
    % Function to calculate pose_error based on projection point to reference point
    
    % Step 1: Create the vector from projection point to reference point
    % This vector points from (X_projection, Y_projection) to (Xref_t, Yref_t)
    projectionpoint2referencepoint = [Xref_t - X_projection, Yref_t - Y_projection];  

    % Step 2: Perform the dot product of the two vectors
    dot_product = dot(projectionpoint2referencepoint, closest2closestplus1);
    
    % Step 3: Calculate the length of the projectionpoint2referencepoint vector
    % The length of the vector is its Euclidean norm
    vector_length = norm(projectionpoint2referencepoint);
    
    % Step 4: Determine pose_error based on the dot product sign
    if dot_product < 0
        pose_error = -vector_length; % Negative length if dot product is negative (ahead of reference point)
    else
        pose_error = vector_length;  % Positive length otherwise (behind reference point)
    end

end
